simulink model "data"  (R2017a)
settings: Solver=FixedStepDiscrete  StartTime=0.0  StopTime=0.1  RelTol=1e-3
libraries: dspswit3 x1, dspindex x1, commutil2 x1
settings Model: Creator=carvalho  LastModifiedBy=carvalho

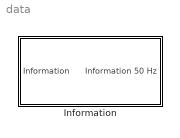
== system data ==
  Information : Subsystem

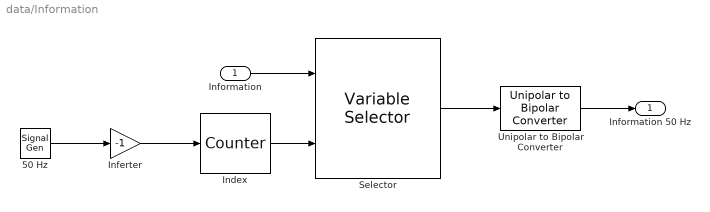
== system data/Information ==
  Information : Inport
  50 Hz : SignalGenerator  WaveForm=square  Frequency=50
  Index : dspswit3/Counter  Direction=Up  CountEvent=Rising edge  CounterSize=32 bits  MaxCount=255  InitialCount=0  Output=Count  HitValue=32  ResetInput=off  SamplesPerFrame=1  Ts=1  CntDtype=double  HitDtype=Logical
  Inferter : Gain  Gain=-1
  Selector : dspindex/Variable Selector  NumInputs=1  rowsOrCols=Columns  IdxMode=Variable  Elements=[1 3]  ZerOneIdxMode=Zero-based  errmode=Clip Index  FillMode=off  FillValues=0
  Unipolar to Bipolar Converter : commutil2/Unipolar to Bipolar Converter  M=2  polarity=Positive  dataType=Inherit via internal rule
      settings: SourceProductName=Communications System Toolbox
  Information 50 Hz : Outport
  wires:
  Unipolar to Bipolar Converter/1 -> Information 50 Hz/1
  Information/1 -> Selector/1
  Selector/1 -> Unipolar to Bipolar Converter/1
  Index/1 -> Selector/2
  Inferter/1 -> Index/1
  50 Hz/1 -> Inferter/1
